simulink model "two_dimention"  (R2022b)
settings: Solver=FixedStepAuto  StartTime=0.0  StopTime=10.0  RelTol=1e-3
libraries: simulink x3
settings Model: Creator=CSPLAB  LastModifiedBy=CSPLAB
settings DataIOCC: ReturnWorkspaceOutputs=off
settings ModelReferenceCC: EnableRefExpFcnMdlSchedulingChecks=on

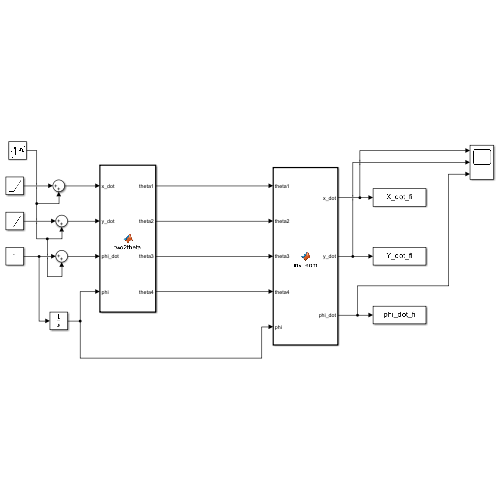
[thumbnail: Simulink's stored preview of the top-level diagram]
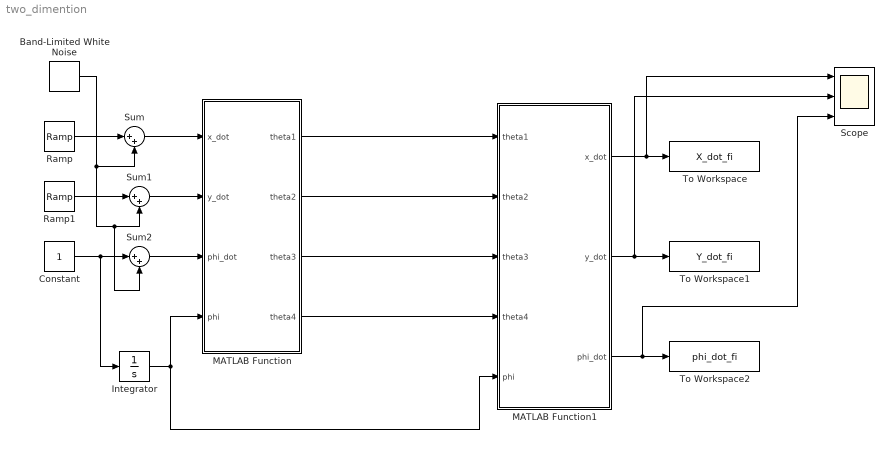
== system two_dimention ==
  Band-Limited White Noise : simulink/Sources/Band-Limited White Noise  Cov=[0.1]  Ts=0.1  seed=[23341]
  Constant : Constant
  Integrator : Integrator
  MATLAB Function : MATLAB Function  TreatAsAtomicUnit=on
  MATLAB Function1 : MATLAB Function  TreatAsAtomicUnit=on
  Ramp : simulink/Sources/Ramp  slope=1  start=0  InitialOutput=0
  Ramp1 : simulink/Sources/Ramp  slope=2  start=0  InitialOutput=0
  Scope : Scope  NumInputPorts=3
  Sum : Sum  Inputs=|++
  Sum1 : Sum  Inputs=|++
  Sum2 : Sum  Inputs=|++
  To Workspace : ToWorkspace  VariableName=X_dot_fi  SaveFormat=Timeseries  SampleTime=-1
  To Workspace1 : ToWorkspace  VariableName=Y_dot_fi  SaveFormat=Timeseries  SampleTime=-1
  To Workspace2 : ToWorkspace  VariableName=phi_dot_fi  SaveFormat=Timeseries  SampleTime=-1
  wires:
  MATLAB Function/1(theta1) -> MATLAB Function1/1(theta1)
  MATLAB Function/2(theta2) -> MATLAB Function1/2(theta2)
  MATLAB Function/3(theta3) -> MATLAB Function1/3(theta3)
  MATLAB Function/4(theta4) -> MATLAB Function1/4(theta4)
  Ramp/1 -> Sum/1
  Constant/1 -> Integrator/1, Sum2/1
  Integrator/1 -> MATLAB Function1/5(phi), MATLAB Function/4(phi)
  MATLAB Function1/1(x_dot) -> Scope/1, To Workspace/1
  MATLAB Function1/2(y_dot) -> Scope/2, To Workspace1/1
  MATLAB Function1/3(phi_dot) -> Scope/3, To Workspace2/1
  Band-Limited White Noise/1 -> Sum2/2, Sum1/2, Sum/2
  Sum/1 -> MATLAB Function/1(x_dot)
  Ramp1/1 -> Sum1/1
  Sum1/1 -> MATLAB Function/2(y_dot)
  Sum2/1 -> MATLAB Function/3(phi_dot)

== matlab function two_dimention/MATLAB Function1 ==
  data: theta1 input; x_dot output; theta2 input; theta3 input; theta4 input; y_dot output; phi_dot output; phi input
function [x_dot, y_dot, phi_dot] = inv_eom(theta1,theta2,theta3,theta4,phi)

    %===== parameter set =====%
    Lx = 0.2375;
    Ly = 0.2394;
    R = 0.05;
    delta = pi/4;


    H = [cos(phi - delta) sin(phi - delta)  -(Lx * sin(delta) + Ly * cos(delta));
         cos(phi + delta) sin(phi + delta)   (Lx * sin(delta) + Ly * cos(delta));
         cos(phi + delta) sin(phi + delta)  -(Lx * sin(delta) + Ly * cos(delta));
         cos(phi - delta) sin(phi - delta)   (Lx * sin(delta) + Ly * cos(delta))];
    A = [R * cos(delta) * theta1,
        R * cos(delta) * theta2,
        R * cos(delta) * theta3,
        R * cos(delta) * theta4];

    X = inv(H' * H) * H' * A;

    x_dot = X(1);
    y_dot = X(2);
    phi_dot = X(3);

== matlab function two_dimention/MATLAB Function ==
  data: x_dot input; theta1 output; y_dot input; phi_dot input; phi input; theta2 output; theta3 output; theta4 output
function [theta1,theta2,theta3,theta4] = two2theta(x_dot, y_dot, phi_dot, phi)
    
    %===== parameter set =====%
    Lx = 0.2375;
    Ly = 0.2394;
    R = 0.05;
    delta = pi/4;

    H = [cos(phi - delta) sin(phi - delta)  -(Lx * sin(delta) + Ly * cos(delta));
         cos(phi + delta) sin(phi + delta)   (Lx * sin(delta) + Ly * cos(delta));
         cos(phi + delta) sin(phi + delta)  -(Lx * sin(delta) + Ly * cos(delta));
         cos(phi - delta) sin(phi - delta)   (Lx * sin(delta) + Ly * cos(delta))];
    X = [x_dot; y_dot; phi_dot];
    A = H * X ./ (R * cos(delta));
    theta1 = A(1, 1);
    theta2 = A(2, 1);
    theta3 = A(3, 1);
    theta4 = A(4, 1);
